simulink model "proyect"  (R2014a)
settings: Solver=ode45  StartTime=0.0  StopTime=15  RelTol=1e-3  EnableMultiTasking=on
settings Model: Creator=Keiver  LastModifiedBy=MS
settings OptimizationCC: SimCompilerOptimization=off
settings DebuggingCC: MergeDetectMultiDrivingBlocksExec=error  FcnCallInpInsideContextMsg=error  FrameProcessingCompatibilityMsg=error  SFExecutionAtInitializationDiag=none
settings HardwareCC: ProdBitPerSizeT=32  ProdBitPerPtrDiffT=32
settings RTWCC: RTWCompilerOptimization=off
settings CodeAppCC: StateflowObjectComments=on
settings ConfigComp: CovMetricSettings=dw  CovHtmlReporting=on  CovSaveCumulativeToWorkspaceVar=on  CovSaveSingleToWorkspaceVar=on  CovExternalEMLEnable=off  CovSFcnEnable=off

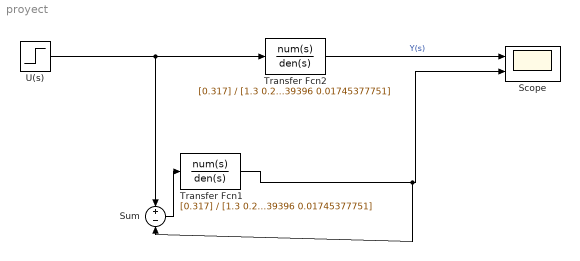
== system proyect ==
  Scope : Scope  NumInputPorts=2
      settings: YMin=-5~-5  YMax=5~5
  Sum : Sum  Inputs=+-
  Transfer Fcn1 : TransferFcn  Numerator=[0.317]  Denominator=[1.3 0.28888 13.2439396 0.01745377751]
  Transfer Fcn2 : TransferFcn  Numerator=[0.317]  Denominator=[1.3 0.28888 13.2439396 0.01745377751]
  U(s) : Step  Time=0  SampleTime=1
  wires:
  U(s)/1 -> Transfer Fcn2/1, Sum/1
  Transfer Fcn2/1 -> Scope/1  "Y(s)"
  Sum/1 -> Transfer Fcn1/1
  Transfer Fcn1/1 -> Sum/2, Scope/2
